simulink model "PubIfDecisionLSM_MDL"  (R2020b)
settings: configuration reference "DspaceConfig" (kept outside this file)
PostLoadFcn:
  | if any(exist('dsrtsu_mdlpostloadfcn', 'file') ~= 0), dsrtsu_mdlpostloadfcn('Execute', bdroot); end
InitFcn:
  | , if any(exist('rtifpga_mdlclblib', 'file') ~= 0), rtifpga_mdlclblib('Init', bdroot); end,
  | , if any(exist('dsmpb_private', 'file') ~= 0), dsmpb_private('dsmpb_mdlclblib', 'Init', bdroot); end,
values from neighbouring files (symbols this model uses):
  P_LSM_ALC_Enable = 0.0    [LSM_Parameter.sldd]
  P_LSM_AwayEdge_offset = 0.1    [LSM_Parameter.sldd]
  P_LSM_CentValidErr = 1.0    [LSM_Parameter.sldd]
  P_LSM_DOP_C0_EN_Limit = 0.8    [LSM_Parameter.sldd]
  P_LSM_DOP_C0_out_Limit = 2.0    [LSM_Parameter.sldd]
  P_LSM_DOP_C1_EN_Limit : value not decoded    [LSM_Parameter.sldd]
  P_LSM_DOP_C1_out_Limit : value not decoded    [LSM_Parameter.sldd]
  P_LSM_DOP_C1AndC2_Lim_X : value not decoded    [LSM_Parameter.sldd]
  P_LSM_DOP_C2_EN_Limit : value not decoded    [LSM_Parameter.sldd]
  P_LSM_DOP_C2_out_Limit : value not decoded    [LSM_Parameter.sldd]
  P_LSM_DOP_In_Pre2Dop_Dis = 1.0    [LSM_Parameter.sldd]
  P_LSM_DOP_Out_Pre2Dop_Dis = 2.0    [LSM_Parameter.sldd]
  P_LSM_DOP_PreDis_X : value not decoded    [LSM_Parameter.sldd]
  P_LSM_DOP_PreDis_Y : value not decoded    [LSM_Parameter.sldd]
  P_LSM_DOPEnableSW = 1.0    [LSM_Parameter.sldd]
  P_LSM_DOPValid_CheckTime = 0.06    [LSM_Parameter.sldd]
  P_LSM_DoubleLine_Curr2Cent_Dislimit = 0.5    [LSM_Parameter.sldd]
  P_LSM_DoubleLine_Dop2Cent_Dislimit = 0.5    [LSM_Parameter.sldd]
  P_LSM_DoubleLine_DOPOut_C1 : value not decoded    [LSM_Parameter.sldd]
  P_LSM_DoubleLine_Pre2Cent_Dislimit = 1.0    [LSM_Parameter.sldd]
  P_LSM_Error_Limit = 0.5    [LSM_Parameter.sldd]
  P_LSM_IFV2CenterAxis = 0.0    [LSM_Parameter.sldd]
  P_LSM_IFV2RearAxis = 0.0    [LSM_Parameter.sldd]
  P_LSM_Line2Edge_limit = 0.5    [LSM_Parameter.sldd]
  P_LSM_Line_Error = 0.1    [LSM_Parameter.sldd]
  P_LSM_LineSTD_Limit = 0.15    [LSM_Parameter.sldd]
  P_LSM_NOH_Switch = 0.0    [LSM_Parameter.sldd]
  P_LSM_OTL_C0_Factor = 1.0    [LSM_Parameter.sldd]
  P_LSM_OTL_C1_Factor = 0.5    [LSM_Parameter.sldd]
  P_LSM_OTL_C2_Factor = 0.5    [LSM_Parameter.sldd]
  P_LSM_Pre2OnlyLineDis = 5.0    [LSM_Parameter.sldd]
  P_LSM_Pre_t = 0.0    [LSM_Parameter.sldd]
  P_LSM_SingleLine_Cent2Edge_Dislimit = 100.0    [LSM_Parameter.sldd]
  P_LSM_SingleLine_Curr2Cent_Dislimit = 0.2    [LSM_Parameter.sldd]
  P_LSM_SingleLine_Dop2Cent_Dislimit = 0.2    [LSM_Parameter.sldd]
  P_LSM_SingleLine_DOPOut_C1 : value not decoded    [LSM_Parameter.sldd]
  P_LSM_SingleLine_Pre2Cent_Dislimit = 0.5    [LSM_Parameter.sldd]
  P_LSM_TJALimitSpd = 60.0    [LSM_Parameter.sldd]
undefined symbols (not defined in the file or in its folder): P_lCS_IFV2CenterAxis, P_LCS_IFV2RearAxis, P_LSM_EntryEdge_offset, P_LSM_EntryLnChngEnSwitch, P_LSM_EntryVanishDis, P_LSM_LinetLostTime, P_LSM_LineWijCal_C12, P_LSM_LineWijCal_C13, P_LSM_MapValid_ErrorSwitch, P_LSM_PosLineLcFac, P_LSM_SpdLim_Stub_Spd, P_LSM_SpdLim_StubLength, P_LSM_SpdTurnAlarm
libraries: simulink x324, TrueDurationTime x11
(part 21 of 25)

== matlab function PubIfDecisionLSM_MDL/Subsystem1/TargetLineCalc_20ms2/TargetLineCalc/NOA ==
  data: LeftEn input boolean size=1; RightEn input boolean size=1; preDis input; RFM_LineL1_Valid input uint8 size=1; RFM_LineL1_A0 input single size=1; RFM_LineL1_A1 input single size=1; RFM_LineL1_A2 input single size=1; RFM_LineL1_A3 input single size=1; RFM_LineL1_Range input single size=1; RFM_LineL2_Valid input uint8 size=1; RFM_LineL2_A0 input single size=1; RFM_LineL2_A1 input single size=1; RFM_LineL2_A2 input single size=1; RFM_LineL2_A3 input single size=1; RFM_LineL2_Range input single size=1; RFM_LineR1_Valid input uint8 size=1; RFM_LineR1_A0 input single size=1; RFM_LineR1_A1 input single size=1; RFM_LineR1_A2 input single size=1; RFM_LineR1_A3 input single size=1; RFM_LineR1_Range input single size=1; RFM_LineR2_Valid input uint8 size=1; RFM_LineR2_A0 input single size=1; RFM_LineR2_A1 input single size=1; RFM_LineR2_A2 input single size=1; RFM_LineR2_A3 input single size=1; RFM_LineR2_Range input single size=1; Exit_Valid input uint8 size=1; Exit_A0 input single size=1; Exit_A1 input single size=1; Exit_A2 input single size=1; Exit_A3 input single size=1; Exit_Range input single size=1; Exit_Start input; Entry_Valid input; Entry_A0 input; Entry_A1 input; Entry_A2 input; Entry_A3 input; Entry_Range input; Entry_Start input; LineRB_Valid input; LineRB_A0 input; LineRB_A1 input; LineRB_A2 input; LineRB_A3 input; LineRB_Range input; LineRB_Start input; RFM_LineCL_Valid input boolean size=1; RFM_LineCL_A0 input single size=1; RFM_LineCL_A1 input single size=1; RFM_LineCL_A2 input single size=1; RFM_LineCL_A3 input single size=1; RFM_LineCL_Range input single size=1; HWASts input uint8 size=1; HWAStsK1 input uint8 size=1; PilotSts input uint8 size=1; LaneChange input uint8 size=1; PilotRoadSts input uint8 size=1; DistanceLim input single size=1; Offset input; kap input; HWALineValid output boolean size=1; MoveIDK1 input int8 size=1; HWALineC3 output single size=1; HWALineC2 output single size=1; HWALineC1 output single size=1; HWALineC0 output single size=1; HWARange output single size=1; HWALeLineValid output boolean size=1; HWALeLineC3 output single size=1; HWALeLineC2 output single size=1; HWALeLineC1 output single size=1; HWALeLineC0 output single size=1; HWALeRange output single size=1; HWARiLineValid output boolean size=1; HWARiLineC3 output single size=1; HWARiLineC2 output single size=1; HWARiLineC1 output single size=1; HWARiLineC0 output single size=1; HWARiRange output single size=1; MoveID output int8 size=1; LockIDK1 input int8 size=1; LockID output int8 size=1; Lock_counterK1 input uint8; Lock_counter output uint8
function [HWALineValid,HWALineC3,HWALineC2,HWALineC1,HWALineC0,HWARange,...
    HWALeLineValid,HWALeLineC3,HWALeLineC2,HWALeLineC1,HWALeLineC0,HWALeRange,...
    HWARiLineValid,HWARiLineC3,HWARiLineC2,HWARiLineC1,HWARiLineC0,HWARiRange,...
    MoveID,LockID,Lock_counter] = fcn(LeftEn,RightEn,preDis,RFM_LineL1_Valid,RFM_LineL1_A0,RFM_LineL1_A1,RFM_LineL1_A2,RFM_LineL1_A3,RFM_LineL1_Range,...
    RFM_LineL2_Valid,RFM_LineL2_A0,RFM_LineL2_A1,RFM_LineL2_A2,RFM_LineL2_A3,RFM_LineL2_Range,...
    RFM_LineR1_Valid,RFM_LineR1_A0,RFM_LineR1_A1,RFM_LineR1_A2,RFM_LineR1_A3,RFM_LineR1_Range,...
    RFM_LineR2_Valid,RFM_LineR2_A0,RFM_LineR2_A1,RFM_LineR2_A2,RFM_LineR2_A3,RFM_LineR2_Range,...
    Exit_Valid,Exit_A0,Exit_A1,Exit_A2,Exit_A3,Exit_Range,Exit_Start,...
    Entry_Valid,Entry_A0,Entry_A1,Entry_A2,Entry_A3,Entry_Range,Entry_Start,...
    LineRB_Valid,LineRB_A0,LineRB_A1,LineRB_A2,LineRB_A3,LineRB_Range,LineRB_Start,...
    RFM_LineCL_Valid,RFM_LineCL_A0,RFM_LineCL_A1,RFM_LineCL_A2,RFM_LineCL_A3,RFM_LineCL_Range,HWASts,HWAStsK1,...
    PilotSts,LaneChange,PilotRoadSts,DistanceLim,Offset,kap,MoveIDK1,LockIDK1,Lock_counterK1)
HWALineValid = false;
HWALineC3 = single(0);
HWALineC2 = single(0);
HWALineC1 = single(0);
HWALineC0 = single(0);
HWARange = single(0);

HWALeLineValid = false;
HWALeLineC3 = single(0);
HWALeLineC2 = single(0);
HWALeLineC1 = single(0);
HWALeLineC0 = single(0);
HWALeRange = single(0);

HWARiLineValid = false;
HWARiLineC3 = single(0);
HWARiLineC2 = single(0);
HWARiLineC1 = single(0);
HWARiLineC0 = single(0);
HWARiRange = single(0);

dy_pre = 0.5*kap*preDis^2;
Curature3_pre = RFM_LineR1_A1 + 2*RFM_LineR1_A2*preDis + 3*RFM_LineR1_A3*(preDis^2);
dy3 = (RFM_LineR1_A0 + RFM_LineR1_A1*preDis + RFM_LineR1_A2*(preDis^2) + RFM_LineR1_A3*(preDis^3) - dy_pre)/sqrt(Curature3_pre^2+single(1));
dyRiRE = (LineRB_A0 + LineRB_A1*preDis + LineRB_A2*(preDis^2) + LineRB_A3*(preDis^3) - dy_pre)/sqrt(Curature3_pre^2+single(1));
RoadWidth_L = (RFM_LineL2_A0-RFM_LineL1_A0)/sqrt(RFM_LineL1_A1^2 + single(1));

MoveID = MoveIDK1;
LockID = LockIDK1;
Lock_counter = max(Lock_counterK1-uint8(1),uint8(0));
if Lock_counter==0
    LockID = int8(0);
end

if (HWASts==1)||(HWASts==7)||(HWASts==0)||HWASts==2
    MoveID = int8(0);
end
Error=false;

%% NOH
if PilotSts~=0
    if HWASts==1||HWASts==2
        if RFM_LineCL_Valid>0
            HWALineValid = true;
            HWALineC3 = RFM_LineCL_A3;
            HWALineC2 = RFM_LineCL_A2;
            HWALineC1 = RFM_LineCL_A1;
            HWALineC0 = RFM_LineCL_A0;
            HWARange = RFM_LineCL_Range;
        end
    end
    if PilotRoadSts==8&&Exit_Valid==1           %汇出（未行驶到汇出线）
        if Exit_Start>30
            HWALineValid = RFM_LineCL_Valid;
            HWALineC3 = RFM_LineCL_A3;
            HWALineC2 = RFM_LineCL_A2;
            HWALineC1 = RFM_LineCL_A1;
            HWALineC0 = RFM_LineCL_A0;
            HWARange = RFM_LineCL_Range;
        elseif Exit_Start>16
            temp_x = [0.5*Exit_Start,Exit_Start,Exit_Start+single(10),Exit_Start+single(30)];
            y1 = RFM_LineCL_A0+RFM_LineCL_A1*temp_x(1)+RFM_LineCL_A2*temp_x(1)^2+RFM_LineCL_A3*temp_x(1)^3;
            y3 = Exit_A0+Exit_A1*temp_x(3)+Exit_A2*temp_x(3)^2+Exit_A3*temp_x(3)^3;
            if y3>0
                y2 = min(1,0.4*y3);
            else
                y2 = max(-1,0.4*y3);
            end
            y4 = Exit_A0+Exit_A1*temp_x(4)+Exit_A2*temp_x(4)^2+Exit_A3*temp_x(4)^3;
            temp_y = [y1,y2,y3,y4];
            [HWALineC3,HWALineC2,HWALineC1,HWALineC0] = pl(temp_x,temp_y);
            HWALineValid = true;
            HWARange = Exit_Start+single(40);
        else
            HWALineValid = true;
            HWALineC3 = Exit_A3;
            HWALineC2 = Exit_A2;
            HWALineC1 = Exit_A1;
            HWALineC0 = Exit_A0;
            HWARange = Exit_Range;
        end
    elseif PilotRoadSts==10&&Exit_Valid==1           %汇出（未行驶到汇出线）
        if preDis<Exit_Start
            HWALineValid = RFM_LineCL_Valid;
            HWALineC3 = RFM_LineCL_A3;
            HWALineC2 = RFM_LineCL_A2;
            HWALineC1 = RFM_LineCL_A1;
            HWALineC0 = RFM_LineCL_A0;
            HWARange = RFM_LineCL_Range;
        else
            HWALineValid = true;
            HWALineC3 = Exit_A3;
            HWALineC2 = Exit_A2;
            HWALineC1 = Exit_A1;
            HWALineC0 = Exit_A0;
            HWARange = Exit_Range;
        end
        
    elseif PilotRoadSts==19&&Exit_Valid==1&&preDis<Exit_Range         % 汇出（行驶到右汇出线）
        HWALineValid = true;
        HWALineC3 = Exit_A3;
        HWALineC2 = Exit_A2;
        HWALineC1 = Exit_A1;
        HWALineC0 = Exit_A0;
        HWARange = Exit_Range;
    elseif PilotRoadSts==19&&Exit_Valid==1&&preDis>=Exit_Range&&(RFM_LineCL_Range-Exit_Range)>20
        temp_x1 = [0.5*Exit_Range,Exit_Range,Exit_Range+single(10),Exit_Range+single(20)];
        y1 = Exit_A0+Exit_A1*temp_x1(1)+Exit_A2*temp_x1(1)^2+Exit_A3*temp_x1(1)^3;
        y2=  Exit_A0+Exit_A1*temp_x1(2)+Exit_A2*temp_x1(2)^2+Exit_A3*temp_x1(2)^3;
        y3 = RFM_LineCL_A0+RFM_LineCL_A1*temp_x1(3)+RFM_LineCL_A2*temp_x1(3)^2+RFM_LineCL_A3*temp_x1(3)^3;
        y4 = RFM_LineCL_A0+RFM_LineCL_A1*temp_x1(4)+RFM_LineCL_A1*temp_x1(4)^2+RFM_LineCL_A1*temp_x1(4)^3;
        temp_y1 = [y1,y2,y3,y4];
        [HWALineC3,HWALineC2,HWALineC1,HWALineC0] = pl(temp_x1,temp_y1);
        HWALineValid = true;
        HWARange = Exit_Range+single(20);
        
    elseif PilotRoadSts==30&&Exit_Valid==1&&preDis<Exit_Range         % 汇出（行驶到左汇出线）
        HWALineValid = true;
        HWALineC3 = Exit_A3;
        HWALineC2 = Exit_A2;
        HWALineC1 = Exit_A1;
        HWALineC0 = Exit_A0;
        HWARange = Exit_Range;
    elseif PilotRoadSts==30&&Exit_Valid==1&&preDis>=Exit_Range&&(RFM_LineCL_Range-Exit_Range)>20
        temp_x1 = [0.5*Exit_Range,Exit_Range,Exit_Range+single(10),Exit_Range+single(20)];
        y1 = Exit_A0+Exit_A1*temp_x1(1)+Exit_A2*temp_x1(1)^2+Exit_A3*temp_x1(1)^3;
        y2=  Exit_A0+Exit_A1*temp_x1(2)+Exit_A2*temp_x1(2)^2+Exit_A3*temp_x1(2)^3;
        y3 = RFM_LineCL_A0+RFM_LineCL_A1*temp_x1(3)+RFM_LineCL_A2*temp_x1(3)^2+RFM_LineCL_A3*temp_x1(3)^3;
        y4 = RFM_LineCL_A0+RFM_LineCL_A1*temp_x1(4)+RFM_LineCL_A1*temp_x1(4)^2+RFM_LineCL_A1*temp_x1(4)^3;
        temp_y1 = [y1,y2,y3,y4];
        [HWALineC3,HWALineC2,HWALineC1,HWALineC0] = pl(temp_x1,temp_y1);
        HWALineValid = true;
        HWARange = Exit_Range+single(20);
    elseif PilotRoadSts==31&&Entry_Valid==1&&LineRB_Valid==1         % 汇出（行驶到右汇出线）
        HWALineValid = true;
        HWALineC3 = Entry_A3;
        HWALineC2 = Entry_A2;
        HWALineC1 = Entry_A1;
        if abs(dyRiRE)>Offset
            HWALineC0 = Entry_A0-0.5*RoadWidth_L-1.2;
        else
            HWALineC0 = LineRB_A0+Offset;
        end
        HWARange = Entry_Range;
  
    

 
    elseif HWASts==3 || HWASts==11 || HWASts==12       %巡航
        MoveID = int8(0);
        if HWAStsK1==5 || HWAStsK1==6
            Lock_counter = uint8(250);
            LockID = int8(0);
        end
        if Lock_counter>0
            if LaneChange==1
                LockID = LockID + int8(1);
            end
            if LaneChange==2
                LockID = LockID - int8(1);
            end
        else
            LockID = int8(0);
        end
        if LockID==1
            if RFM_LineR1_Valid>0&&RFM_LineR2_Valid>0&&...
                    (RFM_LineR1_Range>DistanceLim||RFM_LineR2_Range>DistanceLim)
                HWALineValid = true;
                HWALineC3 = 0.5*(RFM_LineR1_A3+RFM_LineR2_A3);
                HWALineC2 = 0.5*(RFM_LineR1_A2+RFM_LineR2_A2);
                HWALineC1 = 0.5*(RFM_LineR1_A1+RFM_LineR2_A1);
                HWALineC0 = 0.5*(RFM_LineR1_A0+RFM_LineR2_A0);
                HWARange = 0.5*(RFM_LineR1_Range+RFM_LineR2_Range);
            elseif RFM_LineR1_Valid>0&&...
                    RFM_LineR1_Range>DistanceLim
                HWALineValid = true;
                HWALineC3 = RFM_LineR1_A3;
                HWALineC2 = RFM_LineR1_A2;
                HWALineC1 = RFM_LineR1_A1;
                HWALineC0 = RFM_LineR1_A0 - 1.875*sqrt(single(1) + RFM_LineR1_A1*RFM_LineR1_A1);
                HWARange = RFM_LineR1_Range;
            elseif RFM_LineR2_Valid>0&&...
                    RFM_LineR2_Range>DistanceLim
                HWALineValid = true;
                HWALineC3 = RFM_LineR2_A3;
                HWALineC2 = RFM_LineR2_A2;
                HWALineC1 = RFM_LineR2_A1;
                HWALineC0 = RFM_LineR2_A0 + 1.875*sqrt(single(1) + RFM_LineR2_A1*RFM_LineR2_A1);
                HWARange = RFM_LineR2_Range;
            end
        elseif LockID==-1
            if RFM_LineL1_Valid>0&&RFM_LineL2_Valid>0&&...
                    (RFM_LineL1_Range>DistanceLim||RFM_LineL2_Range>DistanceLim)
                HWALineValid = true;
                HWALineC3 = 0.5*(RFM_LineL1_A3+RFM_LineL2_A3);
                HWALineC2 = 0.5*(RFM_LineL1_A2+RFM_LineL2_A2);
                HWALineC1 = 0.5*(RFM_LineL1_A1+RFM_LineL2_A1);
                HWALineC0 = 0.5*(RFM_LineL1_A0+RFM_LineL2_A0);
                HWARange = 0.5*(RFM_LineL1_Range+RFM_LineL2_Range);
            elseif RFM_LineL1_Valid>0&&...
                    RFM_LineL1_Range>DistanceLim
                HWALineValid = true;
                HWALineC3 = RFM_LineL1_A3;
                HWALineC2 = RFM_LineL1_A2;
                HWALineC1 = RFM_LineL1_A1;
                HWALineC0 = RFM_LineL1_A0 - 1.875*sqrt(single(1) + RFM_LineL1_A1*RFM_LineL1_A1);
                HWARange = RFM_LineL1_Range;
            elseif RFM_LineL2_Valid>0&&...
                    RFM_LineL2_Range>DistanceLim
                HWALineValid = true;
                HWALineC3 = RFM_LineL2_A3;
                HWALineC2 = RFM_LineL2_A2;
                HWALineC1 = RFM_LineL2_A1;
                HWALineC0 = RFM_LineL2_A0 + 1.875*sqrt(single(1) + RFM_LineL2_A1*RFM_LineL2_A1);
                HWARange = RFM_LineL2_Range;
            end
        elseif LockID==0
            HWALineValid = RFM_LineCL_Valid;
            HWALineC3 = RFM_LineCL_A3;
            HWALineC2 = RFM_LineCL_A2;
            HWALineC1 = RFM_LineCL_A1;
            HWALineC0 = RFM_LineCL_A0;
            HWARange = RFM_LineCL_Range;
        end
        if RFM_LineL1_Valid>0&&RFM_LineL2_Valid>0&&...
                (RFM_LineL1_Range>DistanceLim||RFM_LineL2_Range>DistanceLim)
%             &&LeftEn
            HWALeLineValid = true;
            HWALeLineC3 = 0.5*(RFM_LineL1_A3+RFM_LineL2_A3);
            HWALeLineC2 = 0.5*(RFM_LineL1_A2+RFM_LineL2_A2);
            HWALeLineC1 = 0.5*(RFM_LineL1_A1+RFM_LineL2_A1);
            HWALeLineC0 = 0.5*(RFM_LineL1_A0+RFM_LineL2_A0);
            HWALeRange = 0.5*(RFM_LineL1_Range+RFM_LineL2_Range);
        end
        if RFM_LineR1_Valid>0&&RFM_LineR2_Valid>0&&...
                (RFM_LineR1_Range>DistanceLim||RFM_LineR2_Range>DistanceLim)
%             &&RightEn
            HWARiLineValid = true;
            HWARiLineC3 = 0.5*(RFM_LineR1_A3+RFM_LineR2_A3);
            HWARiLineC2 = 0.5*(RFM_LineR1_A2+RFM_LineR2_A2);
            HWARiLineC1 = 0.5*(RFM_LineR1_A1+RFM_LineR2_A1);
            HWARiLineC0 = 0.5*(RFM_LineR1_A0+RFM_LineR2_A0);
            HWARiRange = 0.5*(RFM_LineR1_Range+RFM_LineR2_Range);
        end
    elseif HWASts == 5                     %左换道
        if HWAStsK1~=5
            MoveID = MoveID - int8(1);
        end
        if LaneChange==1
            MoveID = MoveID + int8(1);
        end
        if LaneChange==2
            MoveID = MoveID - int8(1);
        end
        if (MoveID>=1)||(MoveID<=-2)
            Error = true;
        end
        if Error==false
            if MoveID==-1
                if RFM_LineL1_Valid>0&&RFM_LineL2_Valid>0&&...
                        (RFM_LineL1_Range>DistanceLim||RFM_LineL2_Range>DistanceLim)
                    HWALineValid = true;
                    HWALineC3 = 0.5*(RFM_LineL1_A3+RFM_LineL2_A3);
                    HWALineC2 = 0.5*(RFM_LineL1_A2+RFM_LineL2_A2);
                    HWALineC1 = 0.5*(RFM_LineL1_A1+RFM_LineL2_A1);
                    HWALineC0 = 0.5*(RFM_LineL1_A0+RFM_LineL2_A0);
                    HWARange = 0.5*(RFM_LineL1_Range+RFM_LineL2_Range);
%                     if LeftEn==1
                        HWALeLineValid = true;
                        HWALeLineC3 = 0.5*(RFM_LineL1_A3+RFM_LineL2_A3);
                        HWALeLineC2 = 0.5*(RFM_LineL1_A2+RFM_LineL2_A2);
                        HWALeLineC1 = 0.5*(RFM_LineL1_A1+RFM_LineL2_A1);
                        HWALeLineC0 = 0.5*(RFM_LineL1_A0+RFM_LineL2_A0);
                        HWALeRange = 0.5*(RFM_LineL1_Range+RFM_LineL2_Range);
%                     end
                elseif RFM_LineL1_Valid>0&&...
                        RFM_LineL1_Range>DistanceLim
                    HWALineValid = true;
                    HWALineC3 = RFM_LineL1_A3;
                    HWALineC2 = RFM_LineL1_A2;
                    HWALineC1 = RFM_LineL1_A1;
                    HWALineC0 = RFM_LineL1_A0 - 1.875*sqrt(single(1) + RFM_LineL1_A1*RFM_LineL1_A1);
                    HWARange = RFM_LineL1_Range;
%                     if LeftEn==1
                        HWALeLineValid = true;
                        HWALeLineC3 = RFM_LineL1_A3;
                        HWALeLineC2 = RFM_LineL1_A2;
                        HWALeLineC1 = RFM_LineL1_A1;
                        HWALeLineC0 = RFM_LineL1_A0 - 1.875*sqrt(single(1) + RFM_LineL1_A1*RFM_LineL1_A1);
                        HWALeRange = RFM_LineL1_Range;
%                     end
                elseif RFM_LineL2_Valid>0&&...
                        RFM_LineL2_Range>DistanceLim
                    HWALineValid = true;
                    HWALineC3 = RFM_LineL2_A3;
                    HWALineC2 = RFM_LineL2_A2;
                    HWALineC1 = RFM_LineL2_A1;
                    HWALineC0 = RFM_LineL2_A0 + 1.875*sqrt(single(1) + RFM_LineL2_A1*RFM_LineL2_A1);
                    HWARange = RFM_LineL2_Range;
%                     if LeftEn==1
                        HWALeLineValid = true;
                        HWALeLineC3 = RFM_LineL2_A3;
                        HWALeLineC2 = RFM_LineL2_A2;
                        HWALeLineC1 = RFM_LineL2_A1;
                        HWALeLineC0 = RFM_LineL2_A0 + 1.875*sqrt(single(1) + RFM_LineL2_A1*RFM_LineL2_A1);
                        HWALeRange = RFM_LineL2_Range;
%                     end
                end
                HWARiLineValid = RFM_LineCL_Valid;
                HWARiLineC3 = RFM_LineCL_A3;
                HWARiLineC2 = RFM_LineCL_A2;
                HWARiLineC1 = RFM_LineCL_A1;
                HWARiLineC0 = RFM_LineCL_A0;
                HWARiRange = RFM_LineCL_Range;
            elseif MoveID==0
                HWALineValid = RFM_LineCL_Valid;
                HWALineC3 = RFM_LineCL_A3;
                HWALineC2 = RFM_LineCL_A2;
                HWALineC1 = RFM_LineCL_A1;
                HWALineC0 = RFM_LineCL_A0;
                HWARange = RFM_LineCL_Range;
            end
        end
    elseif HWASts==6                                     %右换道
        if HWAStsK1~=6
            MoveID = MoveID + int8(1);
        end
        if LaneChange==1
            MoveID = MoveID + int8(1);
        end
        if LaneChange==2
            MoveID = MoveID - int8(1);
        end
        if (MoveID>=2)||(MoveID<=-1)
            Error = true;
        end
        if Error==false
            if MoveID==1
                if RFM_LineR1_Valid>0&&RFM_LineR2_Valid>0&&...
                        (RFM_LineR1_Range>DistanceLim||RFM_LineR2_Range>DistanceLim)
                    HWALineValid = true;
                    HWALineC3 = 0.5*(RFM_LineR1_A3+RFM_LineR2_A3);
                    HWALineC2 = 0.5*(RFM_LineR1_A2+RFM_LineR2_A2);
                    HWALineC1 = 0.5*(RFM_LineR1_A1+RFM_LineR2_A1);
                    HWALineC0 = 0.5*(RFM_LineR1_A0+RFM_LineR2_A0);
                    HWARange = 0.5*(RFM_LineR1_Range+RFM_LineR2_Range);
%                     if RightEn==1
                        HWARiLineValid = true;
                        HWARiLineC3 = 0.5*(RFM_LineR1_A3+RFM_LineR2_A3);
                        HWARiLineC2 = 0.5*(RFM_LineR1_A2+RFM_LineR2_A2);
                        HWARiLineC1 = 0.5*(RFM_LineR1_A1+RFM_LineR2_A1);
                        HWARiLineC0 = 0.5*(RFM_LineR1_A0+RFM_LineR2_A0);
                        HWARiRange = 0.5*(RFM_LineR1_Range+RFM_LineR2_Range);
%                     end
                elseif RFM_LineR1_Valid>0&&...
                        RFM_LineR1_Range>DistanceLim
                    HWALineValid = true;
                    HWALineC3 = RFM_LineR1_A3;
                    HWALineC2 = RFM_LineR1_A2;
                    HWALineC1 = RFM_LineR1_A1;
                    HWALineC0 = RFM_LineR1_A0 - 1.875*sqrt(single(1) + RFM_LineR1_A1*RFM_LineR1_A1);
                    HWARange = RFM_LineR1_Range;
%                     if RightEn==1
                        HWARiLineValid = true;
                        HWARiLineC3 = RFM_LineR1_A3;
                        HWARiLineC2 = RFM_LineR1_A2;
                        HWARiLineC1 = RFM_LineR1_A1;
                        HWARiLineC0 = RFM_LineR1_A0 - 1.875*sqrt(single(1) + RFM_LineR1_A1*RFM_LineR1_A1);
                        HWARiRange = RFM_LineR1_Range;
%                     end
                elseif RFM_LineR2_Valid>0&&...
                        RFM_LineR2_Range>DistanceLim
                    HWALineValid = true;
                    HWALineC3 = RFM_LineR2_A3;
                    HWALineC2 = RFM_LineR2_A2;
                    HWALineC1 = RFM_LineR2_A1;
                    HWALineC0 = RFM_LineR2_A0 + 1.875*sqrt(single(1) + RFM_LineR2_A1*RFM_LineR2_A1);
                    HWARange = RFM_LineR2_Range;
%                     if RightEn==1
                        HWARiLineValid = true;
                        HWARiLineC3 = RFM_LineR2_A3;
                        HWARiLineC2 = RFM_LineR2_A2;
                        HWARiLineC1 = RFM_LineR2_A1;
                        HWARiLineC0 = RFM_LineR2_A0 + 1.875*sqrt(single(1) + RFM_LineR2_A1*RFM_LineR2_A1);
                        HWARiRange = RFM_LineR2_Range;
%                     end
                end
                HWALeLineValid = RFM_LineCL_Valid;
                HWALeLineC3 = RFM_LineCL_A3;
                HWALeLineC2 = RFM_LineCL_A2;
                HWALeLineC1 = RFM_LineCL_A1;
                HWALeLineC0 = RFM_LineCL_A0;
                HWALeRange = RFM_LineCL_Range;
            elseif MoveID==0
                HWALineValid = RFM_LineCL_Valid;
                HWALineC3 = RFM_LineCL_A3;
                HWALineC2 = RFM_LineCL_A2;
                HWALineC1 = RFM_LineCL_A1;
                HWALineC0 = RFM_LineCL_A0;
                HWARange = RFM_LineCL_Range;
            end
        end
    end
end

== matlab function PubIfDecisionLSM_MDL/Subsystem1/TargetLineCalc_20ms2/TargetLineCalc/RoadWidthCalc1 ==
  data: YBranch_b input boolean size=1; VisLineConf input uint8 size=4; a1 input single size=4; a0 input single size=4; LineUpdate input boolean size=1; RoadWidth output single size=1; RoadWidthK1 input single size=1; tLostK1 input single size=1; tLost output single size=1
function [RoadWidth,tLost] = VisRoadWidth(YBranch_b,VisLineConf,a1,a0,LineUpdate,RoadWidthK1,tLostK1)

RoadWidth = RoadWidthK1;
tLost = tLostK1;
Update = false;
temp = single(0);

if LineUpdate
    if (VisLineConf(2)>0)&&(VisLineConf(3)>0)&&(YBranch_b==false)
        if abs(57.3*(atan(a1(2)) - atan(a1(3))))<3
            temp = (a0(2) - a0(3))/sqrt(a1(2)^2 + single(1));
            if (temp>2.5)&&(temp<4.2)
                Update = true;
            end
        end
    end
    if Update
        RoadWidth = 0.1*(temp - RoadWidthK1) + RoadWidthK1;
        tLost = single(0);
    else
        tLost = min(10,tLostK1 + single(0.05));
    end
end

== stateflow chart PubIfDecisionLSM_MDL/Subsystem1/TargetLineCalc_20ms2/TargetLineCalc/Subsystem2/Chart ==
  state Enable
    DopEnable=true;
  state Disable
    DopEnable=false;
  (default) -> Enable
  Enable -> Disable : [Disable==1]
  Disable -> Enable : [Enable==1]
  data: Enable input boolean; DopEnable output boolean; Disable input

== matlab function PubIfDecisionLSM_MDL/Subsystem1/TargetLineCalc_20ms2/TargetLineCalc/Subsystem2/LineSelect1 ==
  data: Off2Cent_flag output; Off2DOP_flag output; Cent2Off_flag output; DOP2Off_flag output; Cent2DOP_flag output; DOP2Cent_flag output uint8; dy_pre output; Y_DOP output; Pre_dis input single; Line_State input; kap input single size=1; LCKSts input; CentLaneValid input boolean size=1; CentLineA3 input single size=1; CentLineA2 input single size=1; CentLineA1 input single size=1; CentLineA0 input single size=1; CentRange input single size=1; aOTL input single size=1; bOTL input single size=1; cOTL input single size=1; dOTL input single size=1; VisEdgeConf input uint8; VisEdgeA3 input single size=2; VisEdgeA2 input single size=2; VisEdgeA1 input single size=2; VisEdgeA0 input single size=2; DoubleLine_Pre2Cent_Dislimit input; DoubleLine_Curr2Cent_Dislimit input; DoubleLine_Dop2Cent_Dislimit input; SingleLine_Cent2Edge_Dislimit input; SingleLine_Pre2Cent_Dislimit input; SingleLine_Curr2Cent_Dislimit input; SingleLine_Dop2Cent_Dislimit input; SingleLine_DOPOut_C1 input; DoubleLine_DOPOut_C1 input; Vehicle_Speed input; DOP_EN input boolean; DOP_OUT input boolean
function [Off2Cent_flag,Off2DOP_flag,Cent2Off_flag,DOP2Off_flag,Cent2DOP_flag,DOP2Cent_flag,dy_pre,Y_DOP]= ...
    LineSelect(Pre_dis,Line_State,kap,LCKSts,...
    CentLaneValid,CentLineA3,CentLineA2,CentLineA1,CentLineA0,CentRange,...
    aOTL,bOTL,cOTL,dOTL,...
    VisEdgeConf,VisEdgeA3,VisEdgeA2,VisEdgeA1,VisEdgeA0,...
    DoubleLine_Pre2Cent_Dislimit,DoubleLine_Curr2Cent_Dislimit,DoubleLine_Dop2Cent_Dislimit,...
    SingleLine_Cent2Edge_Dislimit,SingleLine_Pre2Cent_Dislimit,SingleLine_Curr2Cent_Dislimit,SingleLine_Dop2Cent_Dislimit,...
    SingleLine_DOPOut_C1,DoubleLine_DOPOut_C1,...
    Vehicle_Speed,DOP_EN,DOP_OUT)

DOP2Cent_flag = uint8(0);
Off2Cent_flag=uint8(0);
Off2DOP_flag=uint8(0);
Cent2Off_flag=uint8(0);
DOP2Off_flag=uint8(0);
Cent2DOP_flag=uint8(0);

dy_pre = 0.5*kap*Pre_dis^2;

% CuratureCent_pre = CentLineA1 + 2*CentLineA2*preDis + 3*CentLineA3*(preDis^2);
CuratureDop_pre = cOTL + 2*bOTL*Pre_dis + 3*aOTL*(Pre_dis^2);
Y_Line = CentLineA0+CentLineA1*Pre_dis+CentLineA2*Pre_dis^2+CentLineA3*Pre_dis^3;
Y_DOP = dOTL+cOTL*Pre_dis+bOTL*Pre_dis^2+aOTL*Pre_dis^3;
dyLeRE = (VisEdgeA0(1) + VisEdgeA1(1)*Pre_dis + VisEdgeA2(1)*(Pre_dis^2) + VisEdgeA3(1)*(Pre_dis^3) - dy_pre)/sqrt(CuratureDop_pre^2+single(1));
dyRiRE = (VisEdgeA0(2) + VisEdgeA1(2)*Pre_dis + VisEdgeA2(2)*(Pre_dis^2) + VisEdgeA3(2)*(Pre_dis^3) - dy_pre)/sqrt(CuratureDop_pre^2+single(1));

Error = Y_Line-Y_DOP;
Error2= dy_pre - Y_Line;





%%       DOP到车道线切换    
% DoubleLine_Pre2Cent_Dislimit = 1
% DoubleLine_Curr2Cent_Dislimit = 0.5
% DoubleLine_Dop2Cent_Dislimit =0.5

% SingleLine_Cent2Edge_Dislimit =100

% SingleLine_Pre2Cent_Dislimit = 0.5
% SingleLine_Curr2Cent_Dislimit = 0.2
% SingleLine_Dop2Cent_Dislimit =0.2

if DOP_OUT==1&&Line_State~=0
     DOP2Cent_flag = uint8(1);
elseif DOP_OUT==0
    if Line_State~=24 && Line_State~=25 && Line_State~=0 
        if (abs(Error2)<DoubleLine_Pre2Cent_Dislimit || abs(CentLineA0)<DoubleLine_Curr2Cent_Dislimit || abs(Error)< DoubleLine_Dop2Cent_Dislimit)&&...
                abs(CentLineA1)<DoubleLine_DOPOut_C1
            DOP2Cent_flag = uint8(1);
        end
    else
        if Line_State~=0 
%             if ((VisEdgeConf(1)>=1 && abs(abs(dyLeRE-Y_Line)-abs(VisEdgeA0(1)-CentLineA0))<SingleLine_Cent2Edge_Dislimit)||...
%                     (VisEdgeConf(2)>=1 && abs(abs(dyRiRE-Y_Line)-abs(VisEdgeA0(2)-CentLineA0))<SingleLine_Cent2Edge_Dislimit)) &&...
            if (abs(Error2)<SingleLine_Pre2Cent_Dislimit || abs(CentLineA0)<SingleLine_Curr2Cent_Dislimit || abs(Error)< SingleLine_Dop2Cent_Dislimit)&&...
                    abs(CentLineA1)<SingleLine_DOPOut_C1
                DOP2Cent_flag = uint8(1);
            end
        end

    end
end


%%       OFF到车道线
if  CentLaneValid==true
    Off2Cent_flag=uint8(1);
end
%%       OFF到DOP
if DOP_EN==1 && Vehicle_Speed<55
    Off2DOP_flag=uint8(1);
end
%%       车道线到OFF
if Line_State==0
    Cent2Off_flag=uint8(1);
end
%%       DOP到OFF
if DOP_OUT==1||Vehicle_Speed>=60
    DOP2Off_flag=uint8(1);
end
%%       车道线到DOP
if Line_State==0&&DOP_EN==1&&Vehicle_Speed<55
    Cent2DOP_flag=uint8(1);
end

== matlab function PubIfDecisionLSM_MDL/Subsystem1/TargetLineCalc_20ms2/TargetLineCalc/Subsystem2/MATLAB Function ==
  data: TJA_Line input; DOP_CO input; DOP_C1 input; DOP_C2 input; DOP_CO_EN_Limit input; DOP_C1_EN_Limit input; DOP_C2_EN_Limit input; DOP_CO_out_Limit input; DOP_C1_out_Limit input; DOP_C2_out_Limit input; DOP_In_Pre2Dop_Dis input; DOP_Out_Pre2Dop_Dis input; DOP_Valid input; dy_pre input; Y_DOP input; DOP_In_Enable output boolean; DOP_Out_Enable output
function [DOP_In_Enable,DOP_Out_Enable] = fcn(TJA_Line,DOP_CO,DOP_C1,DOP_C2,DOP_CO_EN_Limit,DOP_C1_EN_Limit,...
    DOP_C2_EN_Limit,DOP_CO_out_Limit,DOP_C1_out_Limit,DOP_C2_out_Limit,DOP_In_Pre2Dop_Dis,DOP_Out_Pre2Dop_Dis,DOP_Valid,dy_pre,Y_DOP)
DOP_In_Enable = false;
DOP_Out_Enable = false;
if TJA_Line~=2 && DOP_Valid>0
    if abs(DOP_CO)<DOP_CO_EN_Limit&&...
            abs(DOP_C1)<DOP_C1_EN_Limit&&...
            abs(DOP_C2)<DOP_C2_EN_Limit&&...
            abs(dy_pre-Y_DOP)<DOP_In_Pre2Dop_Dis
        
        DOP_In_Enable = true;
        
    end
elseif TJA_Line==2
     if abs(DOP_CO)>DOP_CO_out_Limit||...
             abs(DOP_C1)>DOP_C1_out_Limit||...
             abs(DOP_C2)>DOP_C2_out_Limit||...
             abs(dy_pre-Y_DOP)>DOP_Out_Pre2Dop_Dis||...
             DOP_Valid==0
         
        DOP_Out_Enable = true;
        
     end
end

== stateflow chart PubIfDecisionLSM_MDL/Subsystem1/TargetLineCalc_20ms2/TargetLineCalc/Subsystem2/TJA_Line_Select ==
  state OFF
    TJA_Line = uint8(0);
  state DOP_Line
    TJA_Line = uint8(2);
  state EQ4_Line
    TJA_Line = uint8(1);
  (default) -> OFF
  OFF -> DOP_Line [order 2] : [Off2DOP_flag]
  OFF -> EQ4_Line [order 1] : [Off2Cent_flag]
  DOP_Line -> OFF [order 2] : [DOP2Off_flag]
  EQ4_Line -> OFF [order 2] : [Cent2Off_flag]
  EQ4_Line -> DOP_Line [order 1] : [Cent2DOP_flag]
  DOP_Line -> EQ4_Line [order 1] : [DOP2Cent_flag]
  data: TJA_Line output uint8; Cent2Off_flag input; DOP2Cent_flag input; DOP2Off_flag input; Off2Cent_flag input; Off2DOP_flag input; Cent2DOP_flag input

== stateflow chart PubIfDecisionLSM_MDL/Subsystem1/TargetLineCalc_20ms2/TargetLineCalc/Subsystem3/Chart1 ==
  state Name
    PilotTurnSwSts=PilotTurnSwSts_Init;
    m=uint8(0);
    changeVoice=uint8(0);
  state Name1
    en:
    i=0;
    changeVoice=uint8(0);
    m=uint8(1);
    du:
    i=i+1;
    if vehSpd>78&&VehInRightmostLane==1&&nLaneNum>1
    PilotTurnSwSts = uint8(1);
    changeVoice=uint8(1);
    m=uint8(2);
    else
    PilotTurnSwSts=PilotTurnSwSts_Init;
    m=uint8(3);
    end
  state Name2 [commented out]
    PilotTurnSwSts=PilotTurnSwSts_Init;
    en:m=uint8(0);
    changeVoice=uint8(1);
    i=0;
    du:i=i+1;
  (default) -> Name
  Name2 -> ? [commented out] : [i>150]
  Name -> Name1 : [(PilotRoadSts_K==25||...
      | PilotRoadSts_K==26||...
      | PilotRoadSts_K==0)&&...
      | PilotRoadSts==17&&...
      | nLaneNum>1&&...
      | VehInRightmostLane==1]
  Name1 -> Name : [i>500||...
      | PilotRoadSts~=17]
  (default) -> Name2 [commented out] : [(VehInRightmostLane~=1||...
      | nLaneNum<2)&&...
      | m==1]
  Name2 -> ? [commented out] : [(PilotRoadSts_K==25||...
      | PilotRoadSts_K==26)&&...
      | PilotRoadSts==17]
  data: PilotRoadSts input; PilotRoadSts_K input; PilotTurnSwSts_Init input uint8; VehInRightmostLane input; nLaneNum input; vehSpd input; PilotTurnSwSts output uint8; i local; changeVoice output; m output

== matlab function PubIfDecisionLSM_MDL/Subsystem1/TargetLineCalc_20ms2/TargetLineCalc/Subsystem3/EgoLineRef/CalcEgoVehMove ==
  data: dDeltaX output single size=1; tCycle input size=1; Kap input size=1; Vego input size=1; dDeltaY output single size=1; CosOfPsi output single size=1; SinOfPsi output single size=1
function [dDeltaX,dDeltaY,CosOfPsi,SinOfPsi] = EgoVehSts(tCycle,Kap,Vego)
%#codegen

if Kap==0
    dDeltaX = Vego*tCycle;
    dDeltaY = single(0);
    CosOfPsi = single(1);
    SinOfPsi = single(0);
else
    t_Psi = Kap*Vego*tCycle;
    SinOfPsi = sin(t_Psi);
    CosOfPsi = cos(t_Psi);
    dDeltaX = SinOfPsi/Kap;
    dDeltaY = 2*(sin(t_Psi/2)*sin(t_Psi/2))/Kap;
end

== matlab function PubIfDecisionLSM_MDL/Subsystem1/TargetLineCalc_20ms2/TargetLineCalc/Subsystem3/EgoLineRef/CalcEgoVehMove1 ==
  data: EgoLineValid output boolean size=1; Index input uint8 size=1; Dxv input single size=24; Dyv input single size=24; A3 output single size=1; A2 output single size=1; A1 output single size=1; A0 output single size=1; DxMax output single; DxMin output single; TarLineValid input boolean; TarLineA3 input single; TarLineA2 input single; TarLineA1 input single; TarLineA0 input single; LaneChangeEnable output boolean; LaneChangeEnableK1 input boolean
function [EgoLineValid,A3,A2,A1,A0,DxMax,DxMin,LaneChangeEnable] = EgoVehTraj(Index,Dxv,Dyv,TarLineValid,TarLineA3,TarLineA2,TarLineA1,TarLineA0,LaneChangeEnableK1)
%#codegen
LaneChangeEnable = false;
if Index>5
    P = polyfit(Dxv(1:5),Dyv(1:5),3);
    A3 = P(1);
    A2 = P(2);
    A1 = P(3);
    A0 = P(4);
    EgoLineValid = true;
    DxMax = single(0);
    DxMin = Dxv(5);
    if TarLineValid
        if LaneChangeEnableK1==true
            LaneChangeEnable = true;
        else
            t1 = TarLineA3*DxMin^3 + TarLineA2*DxMin^2 + TarLineA1*DxMin + TarLineA0;
            t2 = A3*DxMin^3 + A2*DxMin^2 + A1*DxMin + A0;
            if abs((t1 - t2) - (TarLineA0 - A0))<1
                LaneChangeEnable = true;
            end
        end
    end
else
    EgoLineValid = false;
    A3 = single(0);
    A2 = single(0);
    A1 = single(0);
    A0 = single(0);
    DxMax = single(0);
    DxMin = single(0);
end

== matlab function PubIfDecisionLSM_MDL/Subsystem1/TargetLineCalc_20ms2/TargetLineCalc/Subsystem3/EgoLineRef/P0TrajHistCalc01 ==
  data: EgoDDeltaX input single; EgoDDeltaY input single; EgoCosOfPsi input single; EgoSinOfPsi input single; TrajHistNumK1 input uint8; TrajHistDxvK1 input single; TrajHistDyvK1 input single; TimeK1 input single; CntK1 input uint8; TrajHistNum output uint8; TrajHistDxv output single; TrajHistDyv output single; Time output single; Cnt output uint8
function [TrajHistNum,TrajHistDxv,TrajHistDyv,Time,Cnt]...
    = fcn(EgoDDeltaX,EgoDDeltaY,EgoCosOfPsi,EgoSinOfPsi,...
    TrajHistNumK1,TrajHistDxvK1,TrajHistDyvK1,TimeK1,CntK1)
%#codegen
TrajHistNum = TrajHistNumK1;
TrajHistDxv = TrajHistDxvK1;
TrajHistDyv = TrajHistDyvK1;
Time = TimeK1;
Cnt = CntK1;

if Cnt==0
    TrajHistDxv = single(zeros(24,1));
    TrajHistDyv = single(zeros(24,1));
    Time = single(zeros(24,1));
    TrajHistNum = uint8(1);
    Cnt = uint8(1);
else 
    Temp1 = TrajHistDxv(1) - EgoDDeltaX;
    Temp2 = TrajHistDyv(1) - EgoDDeltaY;
    dDeltaS = Temp1*Temp1 + Temp2*Temp2;
    
    t_AddPosition = (dDeltaS>4);
    t_AddPosition = t_AddPosition&(Time(1)>0.5);
    
    for iBuf=1:TrajHistNum
        dX = TrajHistDxv(iBuf)-EgoDDeltaX;
        dY = TrajHistDyv(iBuf)-EgoDDeltaY;
        TrajHistDxv(iBuf) = dX*EgoCosOfPsi + dY*EgoSinOfPsi;
        TrajHistDyv(iBuf) = -dX*EgoSinOfPsi + dY*EgoCosOfPsi;
        Time(iBuf) = TimeK1(iBuf) + single(0.02);
    end
    if t_AddPosition==true
        TrajHistNum = min(TrajHistNum + uint8(1),uint8(24));
        for iBuf= TrajHistNum:(-1):2
            TrajHistDxv(iBuf) = TrajHistDxv(iBuf-uint8(1));
            TrajHistDyv(iBuf) = TrajHistDyv(iBuf-uint8(1));
            Time(iBuf) = Time(iBuf-uint8(1));
        end
        TrajHistDxv(1) = single(0);
        TrajHistDyv(1) = single(0);
        Time(1) = single(0);
    end
end
end

== stateflow chart PubIfDecisionLSM_MDL/Subsystem1/TargetLineCalc_20ms2/TargetLineCalc/Subsystem3/Subsystem/Chart ==
  state init2
    PilotRoadSts=30;
  state init
    PilotRoadSts=PilotRoadSts_init;
  state init1
    PilotRoadSts=19;
  (default) -> init
  init -> init2 [order 2] : [PilotRoadSts_init==30]
  init2 -> init : [bIsLineExist<2||lExitStub3==1]
  init -> init1 [order 1] : [PilotRoadSts_init==19]
  init1 -> init : [bIsLineExist<2||rExitStub3==1]
  data: PilotRoadSts_init input uint8 size=1; bIsLineExist input uint8 size=1; PilotRoadSts output uint8 size=1; lExitStub3 input boolean size=1; rExitStub3 input boolean size=1
